simulink model "idmdl_2021b"  (R2021b)
settings: Solver=VariableStepAuto  StartTime=0.0  StopTime=100  RelTol=1e-3
undefined symbols (not defined in the file): b, jp, kt, kv, l
libraries: simulink_extras x2
settings Model: Creator=mfussi  LastModifiedBy=mfussi

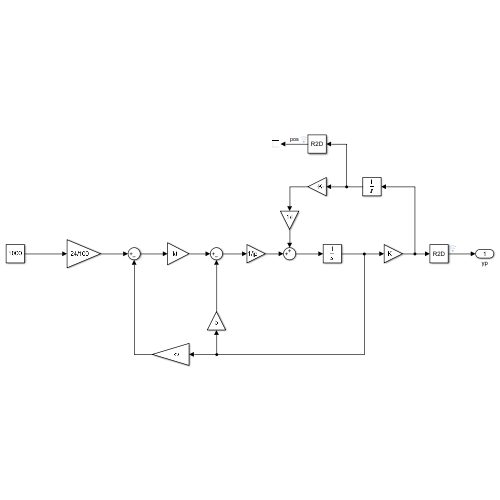
[thumbnail: Simulink's stored preview of the top-level diagram]
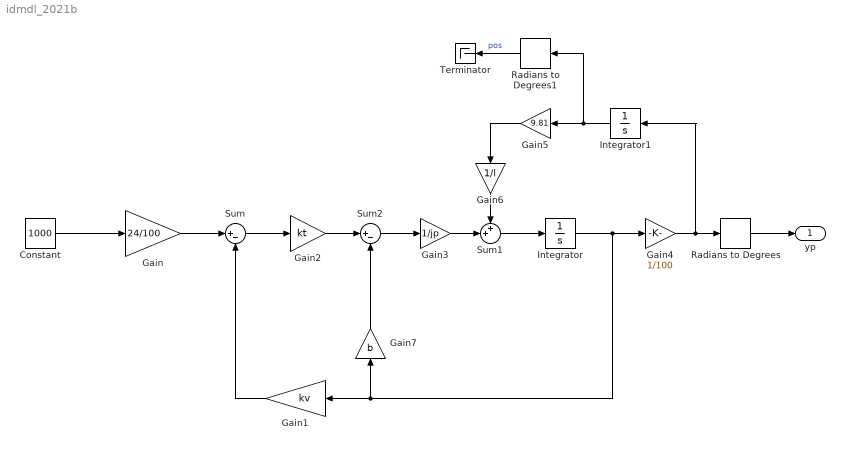
== system idmdl_2021b ==
  Constant : Constant  Value=1000
  Gain : Gain  Gain=24/100
  Gain1 : Gain  Gain=kv
  Gain2 : Gain  Gain=kt
  Gain3 : Gain  Gain=1/jp
  Gain4 : Gain  Gain=1/100
  Gain5 : Gain  Gain=9.81
  Gain6 : Gain  Gain=1/l
  Gain7 : Gain  Gain=b
  Integrator : Integrator
  Integrator1 : Integrator  InitialCondition=pi/2
  Radians to Degrees : simulink_extras/Transformations/Radians to Degrees
  Radians to Degrees1 : simulink_extras/Transformations/Radians to Degrees
  Sum : Sum  Inputs=|+-
  Sum1 : Sum  Inputs=++|
  Sum2 : Sum  Inputs=|+-
  Terminator : Terminator
  yp : Outport
  wires:
  Gain7/1 -> Sum2/2
  Sum2/1 -> Gain3/1
  Sum1/1 -> Integrator/1
  Gain1/1 -> Sum/2
  Gain6/1 -> Sum1/1
  Gain5/1 -> Gain6/1
  Integrator1/1 -> Radians to Degrees1/1, Gain5/1
  Gain3/1 -> Sum1/2
  Integrator/1 -> Gain4/1, Gain1/1, Gain7/1
  Sum/1 -> Gain2/1
  Radians to Degrees/1 -> yp/1
  Gain/1 -> Sum/1
  Gain2/1 -> Sum2/1
  Radians to Degrees1/1 -> Terminator/1  "pos"
  Constant/1 -> Gain/1
  Gain4/1 -> Integrator1/1, Radians to Degrees/1
